simulink model "EEPROMBlocksTemplate"  (Simulink 10.0)
settings: Solver=ode45  StartTime=0.0  StopTime=10.0  RelTol=1e-3  EnableMultiTasking=on
undefined symbols (not defined in the file): CRC32_calc_and_EEPROM_Write_ALL, crc32_calc_intern, EEPROM_Mirror, IO_Blk_Lib_TTC500, IO_EEPROM_GetStatus, IO_EEPROM_Init, IO_EEPROM_Write, Write_Mirror, Write_Mirror_prepare_EEPROM
libraries: simulink x5, IOBlock_Library_TTC580 x2
settings Model: Creator=hokka  LastModifiedBy=hokka
settings DataIOCC: LimitDataPoints=on  SignalLoggingSaveFormat=ModelDataLogs
settings OptimizationCC: ExpressionDepthLimit=2147483647
settings DebuggingCC: SolverPrmCheckMsg=warning  FcnCallInpInsideContextMsg=warning  StateNameClashWarn=warning
settings GRTTargetCC: GeneratePreprocessorConditionals=Disable all
settings ConfigComp: CovExternalEMLEnable=off  CovSFcnEnable=off

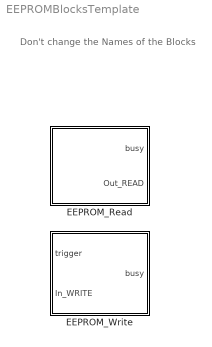
== system EEPROMBlocksTemplate ==
  note: Don't change the Names of the Blocks
  EEPROM_Read : Subsystem  Priority=0  mask(Generated EEPROM_Read){}
      mask help: This Block was generated by the EEPROM Importer
      mask Help:
      | Read out the EEPROM for all given parameters and provide these values on the outports.
      | Reading is done at startup. As long as reading form EEPROM is not terminated for all parameters the busy flag will stay 'true'.
      | CRC_OK will be 0 as long as reading of EEPROM is not completed. Upon success the result is +1. If CRC check fails the result will be -1.
  EEPROM_Write : Subsystem  Priority=0  mask(Generated EEPROM_Write){}
      mask help: This Block was generated by the EEPROM Importer
      mask Help:
      | Aufter receiving the positive edge of a trigger signal the EEPROM_Write - Block will store the parameters into the EEPROM together with the updated CRC32.
      | The busy flag will be 'true' as long as writing to EEPROM is not accomplished or any other EEPROM access is ongoing.
      | The busy flag needs not to be fed back as the trigger rise an internal pending activity as long as EEPROM is not accessible in order to accomplishe the actual writing as soon as the EEPROM is accessible again.

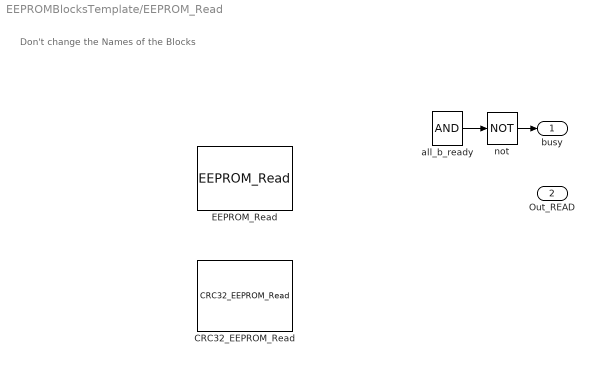
== system EEPROMBlocksTemplate/EEPROM_Read ==
  note: Don't change the Names of the Blocks
  CRC32_EEPROM_Read : IOBlock_Library_TTC580/EEPROM Blocks TTC580 IOlib/CRC32_EEPROM_Read  SampleTime=-1  ttlib=IO_Blk_Lib_TTC500  ttDescription=CRC32_EEPROM_Read  tt_iolib_version=0.26  BasicAddr=0  EndAddr=hex2dec('100')  offset=hex2dec('101')  length=4
      settings: SourceProductName=I/O Blocklibrary for TTC580
  EEPROM_Read : IOBlock_Library_TTC580/EEPROM Blocks TTC580 IOlib/EEPROM_Read  SampleTime=-1  ttlib=IO_Blk_Lib_TTC500  ttDescription=EEPROM_Read  tt_iolib_version=0.26  offset=0  EEPROM_type=uint8
      settings: SourceProductName=I/O Blocklibrary for TTC580
  all_b_ready : Logic  Inputs=1  AllPortsSameDT=off  OutDataTypeStr=boolean
  not : Logic  Operator=NOT  Inputs=1  AllPortsSameDT=off  OutDataTypeStr=boolean
  busy : Outport  VectorParamsAs1DForOutWhenUnconnected=off
  Out_READ : Outport  Port=2  VectorParamsAs1DForOutWhenUnconnected=off
  wires:
  all_b_ready/1 -> not/1
  not/1 -> busy/1

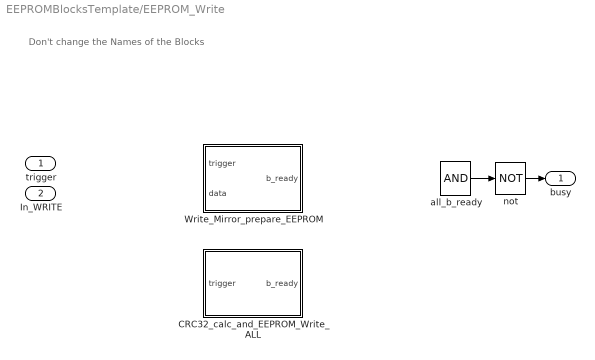
== system EEPROMBlocksTemplate/EEPROM_Write ==
  note: Don't change the Names of the Blocks
  trigger : Inport  OutDataTypeStr=boolean
  In_WRITE : Inport  Port=2
  CRC32_calc_and_EEPROM_Write_ALL : Subsystem  LoadFcn=|  mask(CRC32_calc_and_EEPROM_Write_ALL_Code){SampleTime=-1, ttlib=IO_Blk_Lib_TTC500, ttDescription=CRC32_calc_and_EEPROM_Write_ALL, tt_iolib_version=0.16, BasicAddr=0, EndAddr=hex2dec('100'), offset=hex2dec('101'), length=4}
      | try
      | %
      | %Upgrade Information - standard BEGIN
      | new_color = 'blue';
      | new_ver = '0.16';
      | act_ver = get_param(gcb,'tt_iolib_version');
      | if not(strcmp(act_ver,new_ver))
      |     disp(['Upgrade block: ',gcb,char(10),'       Version: ',act_ver,' -> ',new_ver]);
      |     %switch - case for specific upgrade information e.g. additional parameter required 
      |     %Change appearance and version information
      |     set_param(gcb,'ForegroundColor',new_color);
      |     set_param(gcb,'tt_iolib_version',new_ver);
      | end
      | %Upgrade Information - standard END
      | catch
      | %Standard catch section BEGIN 
      | disp(' ');
      | disp('------------------------------------------------------------');
      | disp('An error occurred in a callback of the TTC580-BlockLib.');
      | disp(['Please check the parameters in the mask of ',gcb]);
      | disp('If you do not encounter any violations, then please '); 
      | disp('copy the following lines and report this to support@ttcontrol.com ');
      | disp('<< begin of error message dump >>');
      | disp(['Version of TTC580-BlockLib: ', get_param(gcb,'tt_iolib_version')]);
      | disp(get_param(gcb,'ttDescription'));
      | disp(gcb);
      | x=lasterror;disp(x.message);
      | disp(get_param(gcb,'MaskValues'));
      | disp(version);
      | disp(computer);
      | disp('<< end of error message dump >>');
      | disp('------------------------------------------------------------');
      | disp(' ');
      | %Standard catch section END
      | end
      mask help:
      | Calculate crc32 for the section [BasicAddr .. EndAddr] out of the EEPROM and write this to a given address (=offset) in EEPROM together with all data in section [BasisAddr .. EndAddr]. This block is supposed to be used within the EEPROM_Importer() only.
      | Note: The trigger input has to be connected to the same trigger as for all EEPROM_Write blocks accessing the interval [BasicAddr .. EndAddr] otherwise data inconsitency may occur.
      mask init:
      | %
      settings: CopyFcn=%deleted
      mask Help: web(which('~.h'))
      mask Callback BasicAddr: %
      mask Callback EndAddr: %
      mask Callback offset: %
      mask Callback length: %
  Write_Mirror_prepare_EEPROM : Subsystem  LoadFcn=|  mask(Write_Mirror_prepare_EEPROM_Code){SampleTime=-1, ttlib=IO_Blk_Lib_TTC500, ttDescription=Write_Mirror_prepare_EEPROM, tt_iolib_version=0.16, offset=0, EEPROM_type=uint8}
      | try
      | %
      | %Upgrade Information - standard BEGIN
      | new_color = 'blue';
      | new_ver = '0.16';
      | act_ver = get_param(gcb,'tt_iolib_version');
      | if not(strcmp(act_ver,new_ver))
      |     disp(['Upgrade block: ',gcb,char(10),'       Version: ',act_ver,' -> ',new_ver]);
      |     %switch - case for specific upgrade information e.g. additional parameter required 
      |     %Change appearance and version information
      |     set_param(gcb,'ForegroundColor',new_color);
      |     set_param(gcb,'tt_iolib_version',new_ver);
      | end
      | %Upgrade Information - standard END
      | catch
      | %Standard catch section BEGIN 
      | disp(' ');
      | disp('------------------------------------------------------------');
      | disp('An error occurred in a callback of the TTC580-BlockLib.');
      | disp(['Please check the parameters in the mask of ',gcb]);
      | disp('If you do not encounter any violations, then please '); 
      | disp('copy the following lines and report this to support@ttcontrol.com ');
      | disp('<< begin of error message dump >>');
      | disp(['Version of TTC580-BlockLib: ', get_param(gcb,'tt_iolib_version')]);
      | disp(get_param(gcb,'ttDescription'));
      | disp(gcb);
      | x=lasterror;disp(x.message);
      | disp(get_param(gcb,'MaskValues'));
      | disp(version);
      | disp(computer);
      | disp('<< end of error message dump >>');
      | disp('------------------------------------------------------------');
      | disp(' ');
      | %Standard catch section END
      | end
      mask help:
      | Write data to the EEPROM_mirror[] in the context of EEPROM_Importer only.
      | Note that offset has to be in the range [0..65535] for TTC580 and [0..32767]for TTC590
      | Note further: No physical IO_EEPROM_Write is perfomted here. This is done in CRC32_calc_and_EEPROM_Write_ALL
      mask init:
      | try
      | switch EEPROM_type 
      |     case {'uint8'}
      |         length = 1; 
      |     case {'uint16'}; 
      |         length = 2; 
      |     case {'uint32'}
      |         length = 4; 
      |     case {'int8'}
      |         length = 1; 
      |     case {'int16'}; 
      |         length = 2; 
      |     case {'int32'}
      |         length = 4; 
      |     case {'single'}
      |         length = 4; 
      |     case {'double'}
      |         length = 8; 
      |     otherwise
      |         error('EEPROM_Write: unsupported type');
      | end
      | 
      | catch
      | %Standard catch section BEGIN 
      | disp(' ');
      | disp('------------------------------------------------------------');
      | disp('An error occurred in a callback of the TTC580-BlockLib.');
      | disp(['Please check the parameters in the mask of ',gcb]);
      | disp('If you do not encounter any violations, then please '); 
      | disp('copy the following lines and report this to support@ttcontrol.com ');
      | disp('<< begin of error message dump >>');
      | disp(['Version of TTC580-BlockLib: ', get_param(gcb,'tt_iolib_version')]);
      | disp(get_param(gcb,'ttDescription'));
      | disp(gcb);
      | x=lasterror;disp(x.message);
      | disp(get_param(gcb,'MaskValues'));
      | disp(version);
      | disp(computer);
      | disp('<< end of error message dump >>');
      | disp('------------------------------------------------------------');
      | disp(' ');
      | %Standard catch section END
      | end
      settings: CopyFcn=%deleted
      mask Help: web(which('~.h'))
      mask Callback offset: %
      mask TypeOptions EEPROM_type: uint8 | uint16 | uint32
      mask Callback EEPROM_type: %
  all_b_ready : Logic  Inputs=1  AllPortsSameDT=off  OutDataTypeStr=boolean
  not : Logic  Operator=NOT  Inputs=1  AllPortsSameDT=off  OutDataTypeStr=boolean
  busy : Outport  VectorParamsAs1DForOutWhenUnconnected=off
  wires:
  all_b_ready/1 -> not/1
  not/1 -> busy/1

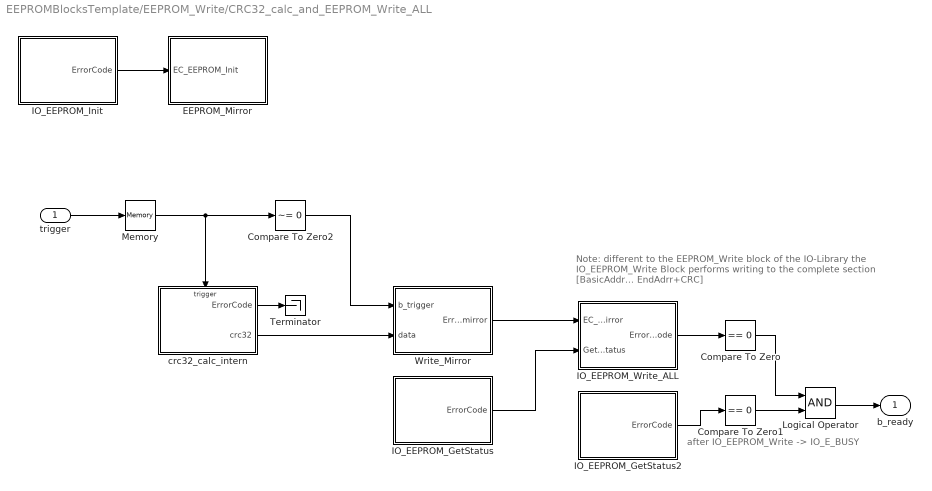
== system EEPROMBlocksTemplate/EEPROM_Write/CRC32_calc_and_EEPROM_Write_ALL ==
  note: Note: different to the EEPROM_Write block
      | of the IO-Library the IO_EEPROM_Write Block
      | performs writing to the complete section [BasicAddr... EndAdrr+CRC]
  note: after IO_EEPROM_Write -> IO_E_BUSY
  trigger : Inport
  Compare To Zero : simulink/Logic and Bit Operations/Compare To Zero  relop===  OutDataTypeStr=boolean  ZeroCross=off
  Compare To Zero1 : simulink/Logic and Bit Operations/Compare To Zero  relop===  OutDataTypeStr=boolean  ZeroCross=off
  Compare To Zero2 : simulink/Logic and Bit Operations/Compare To Zero  relop=~=  OutDataTypeStr=boolean  ZeroCross=off
  EEPROM_Mirror : Subsystem  LoadFcn=|  mask(EEPROM_Mirror_Code){SampleTime=-1, ttlib=IO_Blk_Lib_TTC500, ttDescription=EEPROM_Mirror, tt_iolib_version=0.21, offset=0, length=65536}
      | try
      | %
      | %Upgrade Information - standard BEGIN
      | new_color = 'blue';
      | new_ver = '0.21';
      | act_ver = get_param(gcb,'tt_iolib_version');
      | if not(strcmp(act_ver,new_ver))
      |     disp(['Upgrade block: ',gcb,char(10),'       Version: ',act_ver,' -> ',new_ver]);
      |     %switch - case for specific upgrade information e.g. additional parameter required 
      |     %Change appearance and version information
      |     set_param(gcb,'ForegroundColor',new_color);
      |     set_param(gcb,'tt_iolib_version',new_ver);
      | end
      | %Upgrade Information - standard END
      | catch
      | %Standard catch section BEGIN 
      | disp(' ');
      | disp('------------------------------------------------------------');
      | disp('An error occurred in a callback of the TTC580-BlockLib.');
      | disp(['Please check the parameters in the mask of ',gcb]);
      | disp('If you do not encounter any violations, then please '); 
      | disp('copy the following lines and report this to support@ttcontrol.com ');
      | disp('<< begin of error message dump >>');
      | disp(['Version of TTC580-BlockLib: ', get_param(gcb,'tt_iolib_version')]);
      | disp(get_param(gcb,'ttDescription'));
      | disp(gcb);
      | x=lasterror;disp(x.message);
      | disp(get_param(gcb,'MaskValues'));
      | disp(version);
      | disp(computer);
      | disp('<< end of error message dump >>');
      | disp('------------------------------------------------------------');
      | disp(' ');
      | %Standard catch section END
      | end
      mask help:
      | Read all data from the EEPROM and mirror this onto RAM.
      | The ErrorCode of IO_EEPROM_Init - block must be connected to the input of EEPROM_Mirror.
      | After calling EEPROM_Mirror the global variable EEPROM_mirror is filled and
      | the global variable ErrorCode_EEPROM_mirror contains the returns of IO_EEPROM_Init() and IO_EEPROM_Read().
      mask init:
      | %
      settings: CopyFcn=%deleted
      mask Help: web(which('IO_EEPROM.h'))
      mask Callback offset: %
      mask Callback length: %
  IO_EEPROM_GetStatus : Subsystem  LoadFcn=|  mask(IO_EEPROM_GetStatus_Code){SampleTime=-1, ttlib=IO_Blk_Lib_TTC500, ttDescription=IO_EEPROM_GetStatus, tt_iolib_version=0.19}
      | try
      | %
      | %Upgrade Information - standard BEGIN
      | new_color = 'blue';
      | new_ver = '0.19';
      | act_ver = get_param(gcb,'tt_iolib_version');
      | if not(strcmp(act_ver,new_ver))
      |     disp(['Upgrade block: ',gcb,char(10),'       Version: ',act_ver,' -> ',new_ver]);
      |     %switch - case for specific upgrade information e.g. additional parameter required 
      |     %Change appearance and version information
      |     set_param(gcb,'ForegroundColor',new_color);
      |     set_param(gcb,'tt_iolib_version',new_ver);
      | end
      | %Upgrade Information - standard END
      | catch
      | %Standard catch section BEGIN 
      | disp(' ');
      | disp('------------------------------------------------------------');
      | disp('An error occurred in a callback of the TTC580-BlockLib.');
      | disp('Please copy the following lines and report this to support@tttech.com ');
      | disp('<< begin of error message dump >>');
      | disp(['Version of TTC580-BlockLib: ', get_param(gcb,'tt_iolib_version')]);
      | disp(get_param(gcb,'ttDescription'));
      | disp(gcb);
      | x=lasterror;disp(x.message);
      | disp(get_param(gcb,'MaskValues'));
      | disp(version);
      | disp(computer);
      | disp('<< end of error message dump >>');
      | disp('------------------------------------------------------------');
      | disp(' ');
      | %Standard catch section END
      | end
      mask help: Returns the status of the EEPROM driver.
      mask init:
      | %
      settings: CopyFcn=%deleted
      mask Help: web(which('IO_EEPROM.h'))
  IO_EEPROM_GetStatus2 : Subsystem  LoadFcn=|  mask(IO_EEPROM_GetStatus_Code){SampleTime=-1, ttlib=IO_Blk_Lib_TTC500, ttDescription=IO_EEPROM_GetStatus, tt_iolib_version=0.19}
      | try
      | %
      | %Upgrade Information - standard BEGIN
      | new_color = 'blue';
      | new_ver = '0.19';
      | act_ver = get_param(gcb,'tt_iolib_version');
      | if not(strcmp(act_ver,new_ver))
      |     disp(['Upgrade block: ',gcb,char(10),'       Version: ',act_ver,' -> ',new_ver]);
      |     %switch - case for specific upgrade information e.g. additional parameter required 
      |     %Change appearance and version information
      |     set_param(gcb,'ForegroundColor',new_color);
      |     set_param(gcb,'tt_iolib_version',new_ver);
      | end
      | %Upgrade Information - standard END
      | catch
      | %Standard catch section BEGIN 
      | disp(' ');
      | disp('------------------------------------------------------------');
      | disp('An error occurred in a callback of the TTC580-BlockLib.');
      | disp('Please copy the following lines and report this to support@tttech.com ');
      | disp('<< begin of error message dump >>');
      | disp(['Version of TTC580-BlockLib: ', get_param(gcb,'tt_iolib_version')]);
      | disp(get_param(gcb,'ttDescription'));
      | disp(gcb);
      | x=lasterror;disp(x.message);
      | disp(get_param(gcb,'MaskValues'));
      | disp(version);
      | disp(computer);
      | disp('<< end of error message dump >>');
      | disp('------------------------------------------------------------');
      | disp(' ');
      | %Standard catch section END
      | end
      mask help: Returns the status of the EEPROM driver.
      mask init:
      | %
      settings: CopyFcn=%deleted
      mask Help: web(which('IO_EEPROM.h'))
  IO_EEPROM_Init : Subsystem  LoadFcn=|  mask(IO_EEPROM_Init_Code){SampleTime=-1, ttlib=IO_Blk_Lib_TTC500, ttDescription=IO_EEPROM_Init, tt_iolib_version=0.19}
      | try
      | %
      | %Upgrade Information - standard BEGIN
      | new_color = 'blue';
      | new_ver = '0.19';
      | act_ver = get_param(gcb,'tt_iolib_version');
      | if not(strcmp(act_ver,new_ver))
      |     disp(['Upgrade block: ',gcb,char(10),'       Version: ',act_ver,' -> ',new_ver]);
      |     %switch - case for specific upgrade information e.g. additional parameter required 
      |     %Change appearance and version information
      |     set_param(gcb,'ForegroundColor',new_color);
      |     set_param(gcb,'tt_iolib_version',new_ver);
      | end
      | %Upgrade Information - standard END
      | catch
      | %Standard catch section BEGIN 
      | disp(' ');
      | disp('------------------------------------------------------------');
      | disp('An error occurred in a callback of the TTC580-BlockLib.');
      | disp('Please copy the following lines and report this to support@tttech.com ');
      | disp('<< begin of error message dump >>');
      | disp(['Version of TTC580-BlockLib: ', get_param(gcb,'tt_iolib_version')]);
      | disp(get_param(gcb,'ttDescription'));
      | disp(gcb);
      | x=lasterror;disp(x.message);
      | disp(get_param(gcb,'MaskValues'));
      | disp(version);
      | disp(computer);
      | disp('<< end of error message dump >>');
      | disp('------------------------------------------------------------');
      | disp(' ');
      | %Standard catch section END
      | end
      mask help: Initialization of the EEPROM driver.
      mask init:
      | %
      settings: CopyFcn=%deleted
      mask Help: web(which('IO_EEPROM.h'))
  IO_EEPROM_Write_ALL : Subsystem  LoadFcn=|  mask(IO_EEPROM_Write_Code){SampleTime=-1, ttlib=IO_Blk_Lib_TTC500, ttDescription=IO_EEPROM_Write, tt_iolib_version=0.19, offset=BasicAddr, length=EndAddr-BasicAddr+1+length}
      | try
      | %
      | %Upgrade Information - standard BEGIN
      | new_color = 'blue';
      | new_ver = '0.19';
      | act_ver = get_param(gcb,'tt_iolib_version');
      | if not(strcmp(act_ver,new_ver))
      |     disp(['Upgrade block: ',gcb,char(10),'       Version: ',act_ver,' -> ',new_ver]);
      |     %switch - case for specific upgrade information e.g. additional parameter required 
      |     %Change appearance and version information
      |     set_param(gcb,'ForegroundColor',new_color);
      |     set_param(gcb,'tt_iolib_version',new_ver);
      | end
      | %Upgrade Information - standard END
      | catch
      | %Standard catch section BEGIN 
      | disp(' ');
      | disp('------------------------------------------------------------');
      | disp('An error occurred in a callback of the TTC580-BlockLib.');
      | disp('Please copy the following lines and report this to support@tttech.com ');
      | disp('<< begin of error message dump >>');
      | disp(['Version of TTC580-BlockLib: ', get_param(gcb,'tt_iolib_version')]);
      | disp(get_param(gcb,'ttDescription'));
      | disp(gcb);
      | x=lasterror;disp(x.message);
      | disp(get_param(gcb,'MaskValues'));
      | disp(version);
      | disp(computer);
      | disp('<< end of error message dump >>');
      | disp('------------------------------------------------------------');
      | disp(' ');
      | %Standard catch section END
      | end
      mask help:
      | Copy data from EEPROM_mirror[] to physical EEPROM. Copy activity is triggered by the edge of the input "EC_Write_Mirror" from IO_E_BUSY to IO_E_OK.
      | The output "ErrorCode" is IO_E_BUSY as long as writing to EEPROM is pending. During the activities are performed writing to the physical EEPROM, "ErrorCode" corresponds to the output of the C-driver IO_EEPROM_Write().
      mask init:
      | %
      settings: CopyFcn=%deleted
      mask Help: web(which('IO_EEPROM.h'))
      mask Callback offset: %
      mask Callback length: %
  Logical Operator : Logic  AllPortsSameDT=off  OutDataTypeStr=boolean
  Memory : Memory  LinearizeAsDelay=on
  Terminator : Terminator
  Write_Mirror : Subsystem  LoadFcn=|  mask(Write_Mirror_Code){SampleTime=-1, ttlib=IO_Blk_Lib_TTC500, ttDescription=Write_Mirror, tt_iolib_version=0.19, offset=offset, length=length}
      | try
      | %
      | %Upgrade Information - standard BEGIN
      | new_color = 'blue';
      | new_ver = '0.19';
      | act_ver = get_param(gcb,'tt_iolib_version');
      | if not(strcmp(act_ver,new_ver))
      |     disp(['Upgrade block: ',gcb,char(10),'       Version: ',act_ver,' -> ',new_ver]);
      |     %switch - case for specific upgrade information e.g. additional parameter required 
      |     %Change appearance and version information
      |     set_param(gcb,'ForegroundColor',new_color);
      |     set_param(gcb,'tt_iolib_version',new_ver);
      | end
      | %Upgrade Information - standard END
      | catch
      | %Standard catch section BEGIN 
      | disp(' ');
      | disp('------------------------------------------------------------');
      | disp('An error occurred in a callback of the TTC580-BlockLib.');
      | disp('Please copy the following lines and report this to support@tttech.com ');
      | disp('<< begin of error message dump >>');
      | disp(['Version of TTC580-BlockLib: ', get_param(gcb,'tt_iolib_version')]);
      | disp(get_param(gcb,'ttDescription'));
      | disp(gcb);
      | x=lasterror;disp(x.message);
      | disp(get_param(gcb,'MaskValues'));
      | disp(version);
      | disp(computer);
      | disp('<< end of error message dump >>');
      | disp('------------------------------------------------------------');
      | disp(' ');
      | %Standard catch section END
      | end
      mask help:
      | Write data to the mirror of the EEPROM. ErrorCode is set to IO_E_BUSY for one cycle of writing into EEPROM_mirror[].
      | In case the given data section exceeds given EEPROM boundaries, IO_E_EEPROM_RANGE ErrorCode is returned.
      mask init:
      | %
      settings: CopyFcn=%deleted
      mask Help: web(which('~.h'))
      mask Callback offset: %
      mask Callback length: %
  crc32_calc_intern : Subsystem  LoadFcn=|  mask(crc32_calc_intern_Code){SampleTime=-1, ttlib=IO_Blk_Lib_TTC500, ttDescription=crc32_calc_intern, tt_iolib_version=0.19, EEPROM_mirror=EEPROM_mirror, iBasicAddr_intern=BasicAddr, iEndAddr_intern=EndAddr}
      | try
      | %
      | %Upgrade Information - standard BEGIN
      | new_color = 'blue';
      | new_ver = '0.19';
      | act_ver = get_param(gcb,'tt_iolib_version');
      | if not(strcmp(act_ver,new_ver))
      |     disp(['Upgrade block: ',gcb,char(10),'       Version: ',act_ver,' -> ',new_ver]);
      |     %switch - case for specific upgrade information e.g. additional parameter required 
      |     %Change appearance and version information
      |     set_param(gcb,'ForegroundColor',new_color);
      |     set_param(gcb,'tt_iolib_version',new_ver);
      | end
      | %Upgrade Information - standard END
      | catch
      | %Standard catch section BEGIN 
      | disp(' ');
      | disp('------------------------------------------------------------');
      | disp('An error occurred in a callback of the TTC580-BlockLib.');
      | disp('Please copy the following lines and report this to support@tttech.com ');
      | disp('<< begin of error message dump >>');
      | disp(['Version of TTC580-BlockLib: ', get_param(gcb,'tt_iolib_version')]);
      | disp(get_param(gcb,'ttDescription'));
      | disp(gcb);
      | x=lasterror;disp(x.message);
      | disp(get_param(gcb,'MaskValues'));
      | disp(version);
      | disp(computer);
      | disp('<< end of error message dump >>');
      | disp('------------------------------------------------------------');
      | disp(' ');
      | %Standard catch section END
      | end
      mask help:
      | Calculate crc32 for a section out of the EEPROM.
      | In case the given data section exceeds given EEPROM boundaries, non zero ErrorCode is returned.
      mask init:
      | %
      settings: CopyFcn=%deleted
      mask Help: No further help available for this block
      mask Callback EEPROM_mirror: %
      mask Callback iBasicAddr_intern: %
      mask Callback iEndAddr_intern: %
  b_ready : Outport  VectorParamsAs1DForOutWhenUnconnected=off
  wires:
  Compare To Zero1/1 -> Logical Operator/2
  crc32_calc_intern/1(ErrorCode) -> Terminator/1
  Logical Operator/1 -> b_ready/1
  Compare To Zero/1 -> Logical Operator/1
  Memory/1 -> Compare To Zero2/1, crc32_calc_intern/Trigger
  Compare To Zero2/1 -> Write_Mirror/1(b_trigger)
  crc32_calc_intern/2(crc32) -> Write_Mirror/2(data)
  IO_EEPROM_GetStatus/1(ErrorCode) -> IO_EEPROM_Write_ALL/2(GetStatus)
  Write_Mirror/1(ErrorCode_EEPROM_mirror) -> IO_EEPROM_Write_ALL/1(EC_Write_Mirror)
  trigger/1 -> Memory/1
  IO_EEPROM_Write_ALL/1(ErrorCode) -> Compare To Zero/1
  IO_EEPROM_Init/1(ErrorCode) -> EEPROM_Mirror/1(EC_EEPROM_Init)
  IO_EEPROM_GetStatus2/1(ErrorCode) -> Compare To Zero1/1

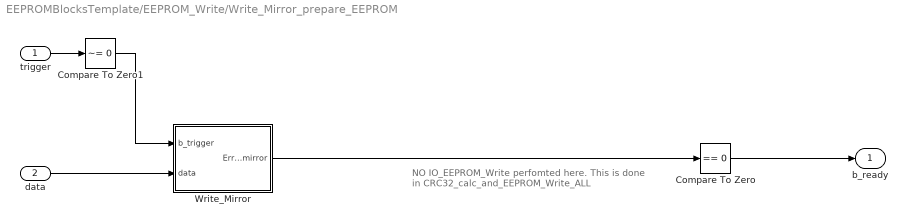
== system EEPROMBlocksTemplate/EEPROM_Write/Write_Mirror_prepare_EEPROM ==
  note: NO IO_EEPROM_Write
      | perfomted here. This is
      | done in CRC32_calc_and_EEPROM_Write_ALL
  trigger : Inport
  data : Inport  Port=2  OutDataTypeStr=EEPROM_type
  Compare To Zero : simulink/Logic and Bit Operations/Compare To Zero  relop===  OutDataTypeStr=boolean  ZeroCross=off
  Compare To Zero1 : simulink/Logic and Bit Operations/Compare To Zero  relop=~=  OutDataTypeStr=boolean  ZeroCross=off
  Write_Mirror : Subsystem  LoadFcn=|  mask(Write_Mirror_Code){SampleTime=-1, ttlib=IO_Blk_Lib_TTC500, ttDescription=Write_Mirror, tt_iolib_version=0.19, offset=offset, length=length}
      | try
      | %
      | %Upgrade Information - standard BEGIN
      | new_color = 'blue';
      | new_ver = '0.19';
      | act_ver = get_param(gcb,'tt_iolib_version');
      | if not(strcmp(act_ver,new_ver))
      |     disp(['Upgrade block: ',gcb,char(10),'       Version: ',act_ver,' -> ',new_ver]);
      |     %switch - case for specific upgrade information e.g. additional parameter required 
      |     %Change appearance and version information
      |     set_param(gcb,'ForegroundColor',new_color);
      |     set_param(gcb,'tt_iolib_version',new_ver);
      | end
      | %Upgrade Information - standard END
      | catch
      | %Standard catch section BEGIN 
      | disp(' ');
      | disp('------------------------------------------------------------');
      | disp('An error occurred in a callback of the TTC580-BlockLib.');
      | disp('Please copy the following lines and report this to support@tttech.com ');
      | disp('<< begin of error message dump >>');
      | disp(['Version of TTC580-BlockLib: ', get_param(gcb,'tt_iolib_version')]);
      | disp(get_param(gcb,'ttDescription'));
      | disp(gcb);
      | x=lasterror;disp(x.message);
      | disp(get_param(gcb,'MaskValues'));
      | disp(version);
      | disp(computer);
      | disp('<< end of error message dump >>');
      | disp('------------------------------------------------------------');
      | disp(' ');
      | %Standard catch section END
      | end
      mask help:
      | Write data to the mirror of the EEPROM. ErrorCode is set to IO_E_BUSY for one cycle of writing into EEPROM_mirror[].
      | In case the given data section exceeds given EEPROM boundaries, IO_E_EEPROM_RANGE ErrorCode is returned.
      mask init:
      | %
      settings: CopyFcn=%deleted
      mask Help: web(which('~.h'))
      mask Callback offset: %
      mask Callback length: %
  b_ready : Outport  VectorParamsAs1DForOutWhenUnconnected=off
  wires:
  Compare To Zero1/1 -> Write_Mirror/1(b_trigger)
  Write_Mirror/1(ErrorCode_EEPROM_mirror) -> Compare To Zero/1
  data/1 -> Write_Mirror/2(data)
  trigger/1 -> Compare To Zero1/1
  Compare To Zero/1 -> b_ready/1

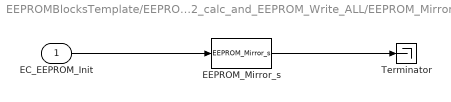
== system EEPROMBlocksTemplate/EEPROM_Write/CRC32_calc_and_EEPROM_Write_ALL/EEPROM_Mirror ==
  EC_EEPROM_Init : Inport
  EEPROM_Mirror_s : S-Function  FunctionName=EEPROM_Mirror_s  Parameters=SampleTime,offset,length  SFunctionDeploymentMode=off  EnableBusSupport=off
  Terminator : Terminator
  wires:
  EC_EEPROM_Init/1 -> EEPROM_Mirror_s/1
  EEPROM_Mirror_s/1 -> Terminator/1

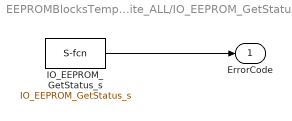
== system EEPROMBlocksTemplate/EEPROM_Write/CRC32_calc_and_EEPROM_Write_ALL/IO_EEPROM_GetStatus ==
  IO_EEPROM_GetStatus_s : S-Function  FunctionName=IO_EEPROM_GetStatus_s  Parameters=SampleTime  SFunctionDeploymentMode=off  EnableBusSupport=off
  ErrorCode : Outport  VectorParamsAs1DForOutWhenUnconnected=off
  wires:
  IO_EEPROM_GetStatus_s/1 -> ErrorCode/1

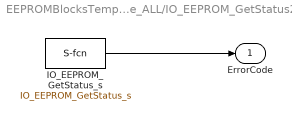
== system EEPROMBlocksTemplate/EEPROM_Write/CRC32_calc_and_EEPROM_Write_ALL/IO_EEPROM_GetStatus2 ==
  IO_EEPROM_GetStatus_s : S-Function  FunctionName=IO_EEPROM_GetStatus_s  Parameters=SampleTime  SFunctionDeploymentMode=off  EnableBusSupport=off
  ErrorCode : Outport  VectorParamsAs1DForOutWhenUnconnected=off
  wires:
  IO_EEPROM_GetStatus_s/1 -> ErrorCode/1

== system EEPROMBlocksTemplate/EEPROM_Write/CRC32_calc_and_EEPROM_Write_ALL/IO_EEPROM_Init ==
  IO_EEPROM_Init_s : S-Function  FunctionName=IO_EEPROM_Init_s  Parameters=SampleTime  SFunctionDeploymentMode=off  EnableBusSupport=off
  ErrorCode : Outport  VectorParamsAs1DForOutWhenUnconnected=off
  wires:
  IO_EEPROM_Init_s/1 -> ErrorCode/1

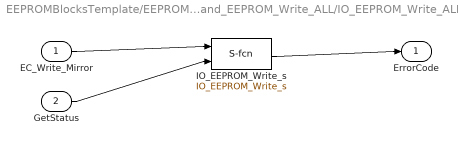
== system EEPROMBlocksTemplate/EEPROM_Write/CRC32_calc_and_EEPROM_Write_ALL/IO_EEPROM_Write_ALL ==
  EC_Write_Mirror : Inport
  GetStatus : Inport  Port=2
  IO_EEPROM_Write_s : S-Function  FunctionName=IO_EEPROM_Write_s  Parameters=SampleTime,offset,length  SFunctionDeploymentMode=off  EnableBusSupport=off
  ErrorCode : Outport  VectorParamsAs1DForOutWhenUnconnected=off
  wires:
  EC_Write_Mirror/1 -> IO_EEPROM_Write_s/1
  GetStatus/1 -> IO_EEPROM_Write_s/2
  IO_EEPROM_Write_s/1 -> ErrorCode/1

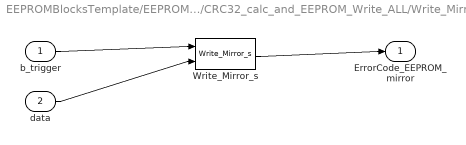
== system EEPROMBlocksTemplate/EEPROM_Write/CRC32_calc_and_EEPROM_Write_ALL/Write_Mirror ==
  b_trigger : Inport
  data : Inport  Port=2
  Write_Mirror_s : S-Function  FunctionName=Write_Mirror_s  Parameters=SampleTime,offset,length  SFunctionDeploymentMode=off  EnableBusSupport=off
  ErrorCode_EEPROM_mirror : Outport  VectorParamsAs1DForOutWhenUnconnected=off
  wires:
  b_trigger/1 -> Write_Mirror_s/1
  data/1 -> Write_Mirror_s/2
  Write_Mirror_s/1 -> ErrorCode_EEPROM_mirror/1

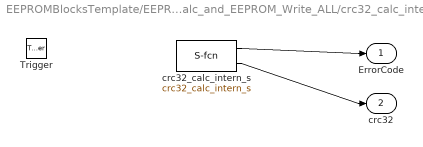
== system EEPROMBlocksTemplate/EEPROM_Write/CRC32_calc_and_EEPROM_Write_ALL/crc32_calc_intern ==
  Trigger : TriggerPort  VariantControl=(inherit)
  crc32_calc_intern_s : S-Function  FunctionName=crc32_calc_intern_s  Parameters=SampleTime,EEPROM_mirror,iBasicAddr_intern,iEndAddr_intern  SFunctionDeploymentMode=off  EnableBusSupport=off
  ErrorCode : Outport  VectorParamsAs1DForOutWhenUnconnected=off
  crc32 : Outport  Port=2  VectorParamsAs1DForOutWhenUnconnected=off
  wires:
  crc32_calc_intern_s/2 -> crc32/1
  crc32_calc_intern_s/1 -> ErrorCode/1

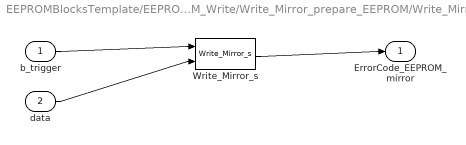
== system EEPROMBlocksTemplate/EEPROM_Write/Write_Mirror_prepare_EEPROM/Write_Mirror ==
  b_trigger : Inport
  data : Inport  Port=2
  Write_Mirror_s : S-Function  FunctionName=Write_Mirror_s  Parameters=SampleTime,offset,length  SFunctionDeploymentMode=off  EnableBusSupport=off
  ErrorCode_EEPROM_mirror : Outport  VectorParamsAs1DForOutWhenUnconnected=off
  wires:
  Write_Mirror_s/1 -> ErrorCode_EEPROM_mirror/1
  data/1 -> Write_Mirror_s/2
  b_trigger/1 -> Write_Mirror_s/1
